simulink model "analogowy"  (R2015a)
settings: Solver=ode45  StartTime=0.0  StopTime=10.0  RelTol=1e-3
undefined symbols (not defined in the file): Id, J, Kp, Kt, Kw, m, psien, Rt, T, TR, Un, uz0, V, wn, Y
settings Model: Creator=Adrian  LastModifiedBy=Adrian

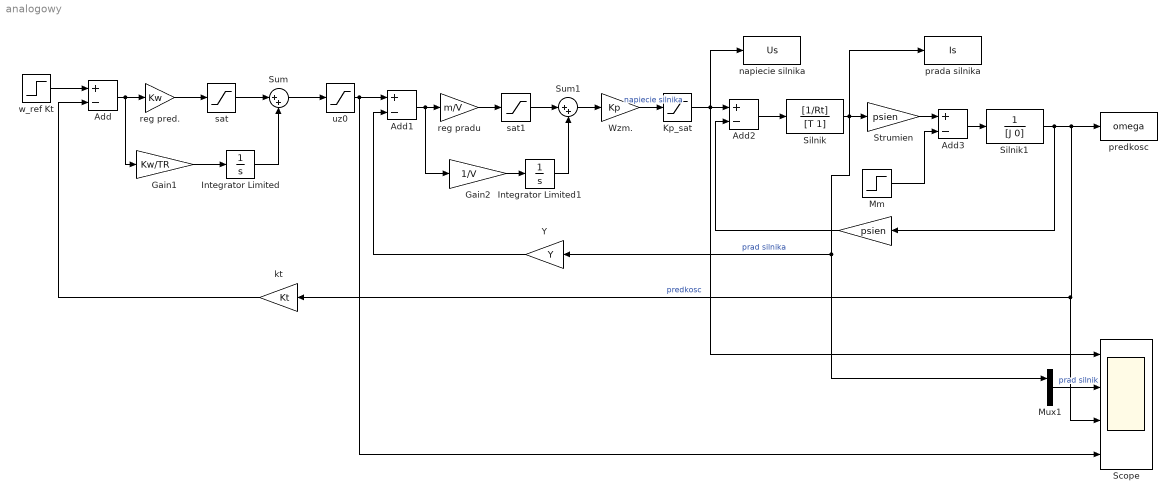
== system analogowy ==
  " " : Gain  Gain=psien
  Add{,1..3} (4 alike) : Sum  Inputs=+-
  Gain1 : Gain  Gain=Kw/TR
  Gain2 : Gain  Gain=1/V
  Integrator Limited : Integrator  LimitOutput=on  UpperSaturationLimit=1  LowerSaturationLimit=0
  Integrator Limited1 : Integrator  LimitOutput=on  UpperSaturationLimit=1  LowerSaturationLimit=0
  Kp_sat : Saturate
  Mm : Step  After=J  SampleTime=0
  Mux1 : Mux  Inputs=2
  Scope : Scope  NumInputPorts=4
      settings: YMin=-5~-5~-5~-5  YMax=5~5~5~5
  Silnik : TransferFcn  Numerator=[1/Rt]  Denominator=[T 1]
  Silnik1 : TransferFcn  Denominator=[J 0]
  Strumien : Gain  Gain=psien
  Sum : Sum  Inputs=|++
  Sum1 : Sum  Inputs=|++
  Wzm. : Gain  Gain=Kp
  Y : Gain  Gain=Y
  kt : Gain  Gain=Kt
  napiecie silnika : ToWorkspace  VariableName=Us  SaveFormat=Timeseries  SampleTime=-1
  prada silnika : ToWorkspace  VariableName=Is  SaveFormat=Timeseries  SampleTime=-1
  predkosc : ToWorkspace  VariableName=omega  SaveFormat=Timeseries  SampleTime=-1
  reg pradu : Gain  Gain=m/V
  reg pred. : Gain  Gain=Kw
  sat : Saturate  UpperLimit=wn
  sat1 : Saturate  UpperLimit=Id
  uz0 : Saturate  UpperLimit=uz0
  w_ref Kt : Step  After=Un  SampleTime=0
  wires:
  Sum/1 -> uz0/1
  w_ref Kt/1 -> Add/1
  Add/1 -> reg pred./1, Gain1/1
  kt/1 -> Add/2
  reg pred./1 -> sat/1
  sat/1 -> Sum/1
  Gain1/1 -> Integrator Limited/1
  Integrator Limited/1 -> Sum/2
  Add1/1 -> Gain2/1, reg pradu/1
  reg pradu/1 -> sat1/1
  sat1/1 -> Sum1/1
  Gain2/1 -> Integrator Limited1/1
  Integrator Limited1/1 -> Sum1/2
  Sum1/1 -> Wzm./1
  Add2/1 -> Silnik/1
  Wzm./1 -> Kp_sat/1  "napiecie silnika"
  Strumien/1 -> Add3/1
  Add3/1 -> Silnik1/1
  " "/1 -> Add2/2
  Y/1 -> Add1/2
  Silnik/1 -> Mux1/1, Y/1, prada silnika/1, Strumien/1  "prad silnika"
  Mux1/1 -> Scope/2  "prad silnik"
  Silnik1/1 -> " "/1, Scope/3, kt/1, predkosc/1  "predkosc"
  uz0/1 -> Scope/4, Add1/1
  Mm/1 -> Add3/2
  Kp_sat/1 -> Scope/1, napiecie silnika/1, Add2/1
